simulink model "runStepperMotor_TestBench"  (R2026a)
settings: Solver=VariableStepAuto  StopTime=1
settings Model: Creator=drew  LastModifiedBy=drew

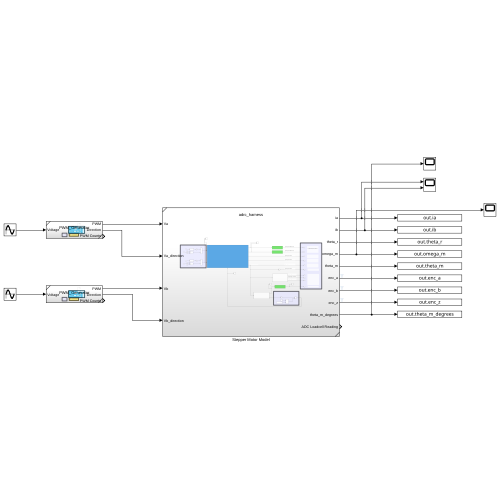
[thumbnail: Simulink's stored preview of the top-level diagram]
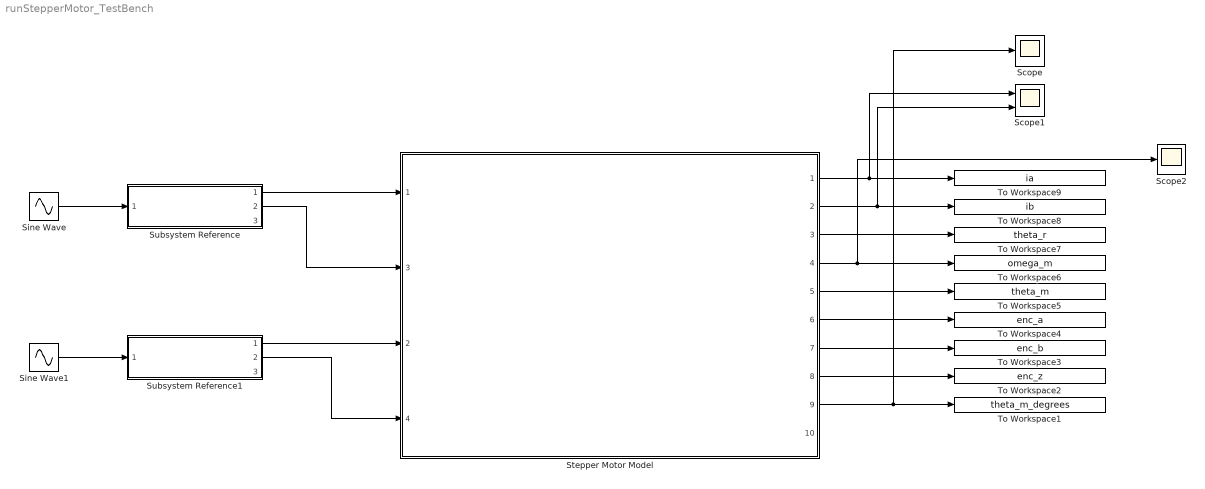
== system runStepperMotor_TestBench ==
  Scope : Scope
      settings: Title=Rotor Position  ActiveDisplayYMinimum=-3.943898562572361  ActiveDisplayYMaximum=3.7218332481541276  DataLoggingVariableName=ScopeData5
  Scope1 : Scope  NumInputPorts=2
      settings: Title=Stepper Motor Current  ActiveDisplayYMinimum=-8191.8749999999982  ActiveDisplayYMaximum=73726.875  DataLoggingVariableName=ScopeData7
  Scope2 : Scope
      settings: ActiveDisplayYMinimum=-76.106104627527571  ActiveDisplayYMaximum=77.05696550033926  DataLoggingVariableName=ScopeData12
  Sine Wave : Sin  Amplitude=48  Frequency=2*pi*50  SampleTime=0
  Sine Wave1 : Sin  Amplitude=48  Frequency=2*pi*50  Phase=-pi/2  SampleTime=0
  Stepper Motor Model : Subsystem  ReferencedSubsystem=adrc_harness
      settings: PortSchema="{\"entries\":[{\"content\":{\"sides\":[{\"content\":{\"connectorIds\":[\"In1\",\"In3\",\"In2\",\"In4\"]},\"type\":\"ConnectorPlacement.EquallySpacedRectSide\",\"uuid\":\"db952c66-fc57-447a-862c-b79330cada38\"},{\"content\":{\"connectorIds\":[\"Out1\",\"Out2\",\"Out3\",\"Out4\",\"Out5\",\"Out6\",\"Out7\",\"Out8\",\"Out9\",\"Out10\"],\"side\":\"RIGHT\"},\"type\":\"ConnectorPlacement.EquallySpacedRectSide\",\"uuid\":\"12562dc1-b5c4-4239-b729-963395de8428\"},{\"content\":{\"side\":\"TOP\"},\"type\":\"ConnectorPlacement.EquallySpacedRectSide\",\"uuid\":\"3dbdfbee-8cdb-483e-891a-ab3c030ef055\"}]},\"type\":\"ConnectorPlacement.EquallySpacedConnector\",\"uuid\":\"9d79cb43-5fdf-4c5b-b972-7a6fb554b8ba\"}],\"packageUris\":[\"http://schema.mathworks.com/mf0/Connector/R2020b\"],\"version\":\"1.0\"}"
  Subsystem Reference : Subsystem  ReferencedSubsystem=PWM_Generator
  Subsystem Reference1 : Subsystem  ReferencedSubsystem=PWM_Generator
  To Workspace1 : ToWorkspace  VariableName=theta_m_degrees  SaveFormat=Structure With Time  SampleTime=-1
  To Workspace2 : ToWorkspace  VariableName=enc_z  SaveFormat=Structure With Time  SampleTime=-1
  To Workspace3 : ToWorkspace  VariableName=enc_b  SaveFormat=Structure With Time  SampleTime=-1
  To Workspace4 : ToWorkspace  VariableName=enc_a  SaveFormat=Structure With Time  SampleTime=-1
  To Workspace5 : ToWorkspace  VariableName=theta_m  SaveFormat=Structure With Time  SampleTime=-1
  To Workspace6 : ToWorkspace  VariableName=omega_m  SaveFormat=Structure With Time  SampleTime=-1
  To Workspace7 : ToWorkspace  VariableName=theta_r  SaveFormat=Structure With Time  SampleTime=-1
  To Workspace8 : ToWorkspace  VariableName=ib  SaveFormat=Structure With Time  SampleTime=-1
  To Workspace9 : ToWorkspace  VariableName=ia  SaveFormat=Structure With Time  SampleTime=-1
  wires:
  Sine Wave1/1 -> Subsystem Reference1/1
  Sine Wave/1 -> Subsystem Reference/1
  Stepper Motor Model/9 -> Scope/1, To Workspace1/1
  Stepper Motor Model/8 -> To Workspace2/1
  Stepper Motor Model/7 -> To Workspace3/1
  Stepper Motor Model/6 -> To Workspace4/1
  Stepper Motor Model/5 -> To Workspace5/1
  Stepper Motor Model/4 -> Scope2/1, To Workspace6/1
  Stepper Motor Model/1 -> Scope1/1, To Workspace9/1
  Stepper Motor Model/2 -> Scope1/2, To Workspace8/1
  Stepper Motor Model/3 -> To Workspace7/1
  Subsystem Reference/1 -> Stepper Motor Model/1
  Subsystem Reference/2 -> Stepper Motor Model/3
  Subsystem Reference1/1 -> Stepper Motor Model/2
  Subsystem Reference1/2 -> Stepper Motor Model/4
